simulink model "SignalGen_tx"  (R2016a)
settings: Solver=VariableStepAuto  StartTime=0.0  StopTime=inf  RelTol=1e-3
libraries: c2000scilib x2
settings Model: Creator=skelter_win  LastModifiedBy=skelter_win

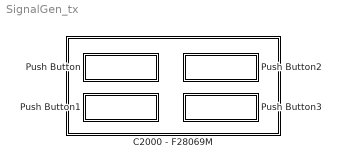
== system SignalGen_tx ==
  C2000 - F28069M : Subsystem
  Push Button : Subsystem  DialogController=hmiCreateDDGDialog  IsWebBlock=on  mask(MWDashboardBlock){webBlockId=04a03bbf-e288-419a-9aa2-a1d98a8ac23b, webBlockType=pushbutton, ShowInLibBrwoser=on, ShowInitialText=on, HMISrcModelName=SignalGen_tx}
      mask prompts: webBlockId "WebBlock Id"; webBlockType "WebBlock Type"; HMISrcModelName "Source Model"
      mask Help: helpview([docroot '/mapfiles/simulink.map'], 'hmi_push_button')
      mask Display:
      | model = bdroot(gcb);
      | if strcmp(get_param(model,'BlockDiagramType'), 'library')
      |     image([(matlabroot) '/toolbox/simulink/hmi/icons/PushButton.png']);
      | end
  Push Button1 : Subsystem  DialogController=hmiCreateDDGDialog  IsWebBlock=on  mask(MWDashboardBlock){webBlockId=627a02fb-e01a-465c-a061-31904469fec2, webBlockType=pushbutton, ShowInLibBrwoser=on, ShowInitialText=on, HMISrcModelName=SignalGen_tx}
      mask prompts: webBlockId "WebBlock Id"; webBlockType "WebBlock Type"; HMISrcModelName "Source Model"
      mask Help: helpview([docroot '/mapfiles/simulink.map'], 'hmi_push_button')
      mask Display:
      | model = bdroot(gcb);
      | if strcmp(get_param(model,'BlockDiagramType'), 'library')
      |     image([(matlabroot) '/toolbox/simulink/hmi/icons/PushButton.png']);
      | end
  Push Button2 : Subsystem  DialogController=hmiCreateDDGDialog  IsWebBlock=on  mask(MWDashboardBlock){webBlockId=61bc546c-6ead-4c2e-b435-9c05180ef064, webBlockType=pushbutton, ShowInLibBrwoser=on, ShowInitialText=on, HMISrcModelName=SignalGen_tx}
      mask prompts: webBlockId "WebBlock Id"; webBlockType "WebBlock Type"; HMISrcModelName "Source Model"
      mask Help: helpview([docroot '/mapfiles/simulink.map'], 'hmi_push_button')
      mask Display:
      | model = bdroot(gcb);
      | if strcmp(get_param(model,'BlockDiagramType'), 'library')
      |     image([(matlabroot) '/toolbox/simulink/hmi/icons/PushButton.png']);
      | end
  Push Button3 : Subsystem  DialogController=hmiCreateDDGDialog  IsWebBlock=on  mask(MWDashboardBlock){webBlockId=b2d2cfc0-730b-4de7-9bea-d454c58a51bc, webBlockType=pushbutton, ShowInLibBrwoser=on, ShowInitialText=on, HMISrcModelName=SignalGen_tx}
      mask prompts: webBlockId "WebBlock Id"; webBlockType "WebBlock Type"; HMISrcModelName "Source Model"
      mask Help: helpview([docroot '/mapfiles/simulink.map'], 'hmi_push_button')
      mask Display:
      | model = bdroot(gcb);
      | if strcmp(get_param(model,'BlockDiagramType'), 'library')
      |     image([(matlabroot) '/toolbox/simulink/hmi/icons/PushButton.png']);
      | end

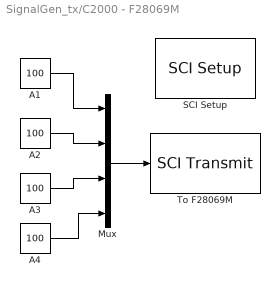
== system SignalGen_tx/C2000 - F28069M ==
  A{1..4} (4 alike) : Constant  Value=100  OutDataTypeStr=uint8
  Mux : Mux
  SCI Setup : c2000scilib/SCI Setup  Priority=-99  commModeA=protocol  baudRateA=115200  charLenA=8  stopBitA=1  parityA=none  timeoutA=1.0  commModeB=raw data  baudRateB=115200  charLenB=8  stopBitB=1  parityB=none  timeoutB=1.0  commModeC=raw data  baudRateC=115200  charLenC=8  stopBitC=1  parityC=none  timeoutC=1.0  commModeD=protocol  baudRateD=115200  charLenD=8  stopBitD=1  parityD=none  timeoutD=1.0
  To F28069M : c2000scilib/SCI Transmit  module=COM 2  header='S'  tail='E'
  wires:
  Mux/1 -> To F28069M/1
  A1/1 -> Mux/1
  A2/1 -> Mux/2
  A4/1 -> Mux/4
  A3/1 -> Mux/3

== system SignalGen_tx/Push Button ==

== system SignalGen_tx/Push Button1 ==

== system SignalGen_tx/Push Button2 ==

== system SignalGen_tx/Push Button3 ==
